simulink model "Due_Test"  (R2020a)
settings: Solver=FixedStepAuto  StartTime=0.0  StopTime=inf  FixedStep=T  RelTol=1e-3  EnableMultiTasking=on
undefined symbols (not defined in the file): Iumax, T, wmax
libraries: arduinolib x6, eeStairGenerator x1
settings Model: SILPILModeSetting=veronly  ExtModeTrigDuration=2  Creator=Nguyen Tung  LastModifiedBy=Nguyen Tung
settings OptimizationCC: StrengthReduction=on  PassReuseOutputArgsAs=Individual arguments  ZeroExternalMemoryAtStartup=off  ZeroInternalMemoryAtStartup=off  MaxStackSize=64  OptimizeBlockOrder=speed  OptimizationPriority=Speed  OptimizationCustomize=off  MultiThreadedLoops=on  EfficientTunableParamExpr=on
settings DebuggingCC: ParameterTunabilityLossMsg=error
settings HardwareCC: ProdBitPerPointer=32  ProdBitPerSizeT=32  ProdBitPerPtrDiffT=32  ProdLargestAtomicInteger=Long  ProdLargestAtomicFloat=Double  ProdWordSize=32  ProdHWDeviceType=ARM Compatible->ARM Cortex
settings SFSimCC: MATLABDynamicMemAlloc=off
settings RTWCC: SystemTargetFile=ert.tlc  HardwareBoard=Arduino Due  TLCOptions=-aInlineSetEventsForThisBaseRateFcn=TLC_FALSE -aSuppressMultiTaskScheduler=TLC_FALSE -aRateBasedStepFcn=1  TemplateMakefile=ert_default_tmf  GenerateReport=on  Toolchain=Arduino ARM  BuildConfiguration=Faster Runs
settings CodeAppCC: ForceParamTrailComments=on  IgnoreCustomStorageClasses=off  OperatorAnnotations=on  SimulinkDataObjDesc=on  SFDataObjDesc=on  InsertBlockDesc=on
settings ERTTargetCC: SupportContinuousTime=on  SupportVariableSizeSignals=on  ExtModeStaticAllocSize=20000

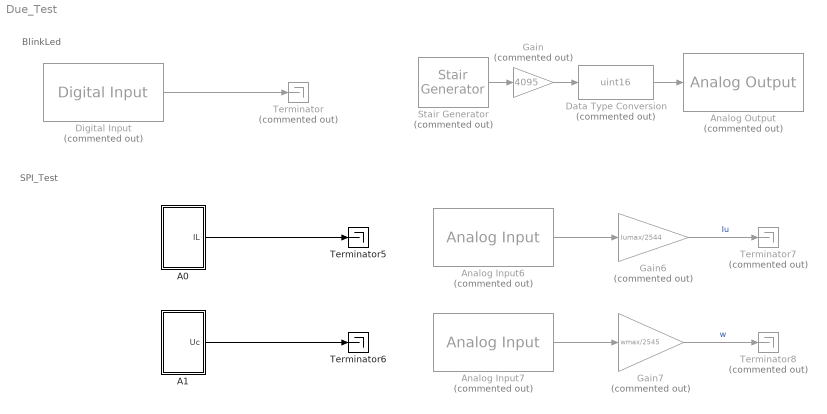
== system Due_Test ==
  note: SPI_Test
  note: BlinkLed
  A0 : Subsystem
  A1 : Subsystem
  Analog Input6 : arduinolib/Analog Input  Commented=on  pinNumber=2  ReadResultsOnly=off  ConversionTriggerSource=Software  ExternalTriggerType=uint32( 0 )  OutputDataType=uint16  EnableConversionCompleteNotify=off  EnableOuputStatus=off  SampleTime=T  blockPlatform=arduino
  Analog Input7 : arduinolib/Analog Input  Commented=on  pinNumber=3  ReadResultsOnly=off  ConversionTriggerSource=Software  ExternalTriggerType=uint32( 0 )  OutputDataType=uint16  EnableConversionCompleteNotify=off  EnableOuputStatus=off  SampleTime=T  blockPlatform=arduino
  Analog Output : arduinolib/Analog Output  Commented=on  DACpin=DAC1  blockPlatform=arduino
      settings: SourceProductBaseCode=ARDUINO
  Data Type Conversion : DataTypeConversion  Commented=on  OutDataTypeStr=uint16
  Digital Input : arduinolib/Digital Input  Commented=on  pinNumber=8  Direction=input  SampleTime=T  blockPlatform=arduino
  Gain : Gain  Commented=on  Gain=4095
  Gain6 : Gain  Commented=on  Gain=Iumax/2544
  Gain7 : Gain  Commented=on  Gain=wmax/2545
  Stair Generator : eeStairGenerator/Stair Generator  Commented=on  LabelModeActiveChoice=Discrete  TimeInput=[5 10 15 20 25 30 35]  AmplitudeInput=[0 0.2 0.4 0.6 0.8 1 0]  SampleTime=T  RepeatPattern=on  OutDataTypeStr=double
      settings: SourceProductBaseCode=PS
  Terminator : Terminator  Commented=on
  Terminator5 : Terminator
  Terminator6 : Terminator
  Terminator7 : Terminator  Commented=on
  Terminator8 : Terminator  Commented=on
  wires:
  Digital Input/1 -> Terminator/1
  Gain7/1 -> Terminator8/1  "w"
  Gain6/1 -> Terminator7/1  "Iu"
  Analog Input7/1 -> Gain7/1
  Analog Input6/1 -> Gain6/1
  Stair Generator/1 -> Gain/1
  Data Type Conversion/1 -> Analog Output/1
  Gain/1 -> Data Type Conversion/1
  A0/1(IL) -> Terminator5/1
  A1/1(Uc) -> Terminator6/1

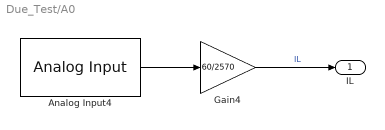
== system Due_Test/A0 ==
  Analog Input4 : arduinolib/Analog Input  pinNumber=0  ReadResultsOnly=off  ConversionTriggerSource=Software  ExternalTriggerType=uint32( 0 )  OutputDataType=uint16  EnableConversionCompleteNotify=off  EnableOuputStatus=off  SampleTime=T  blockPlatform=arduino
  Gain4 : Gain  Gain=60/2570
  IL : Outport
  wires:
  Analog Input4/1 -> Gain4/1
  Gain4/1 -> IL/1  "IL"

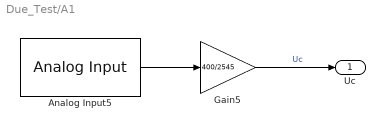
== system Due_Test/A1 ==
  Analog Input5 : arduinolib/Analog Input  pinNumber=1  ReadResultsOnly=off  ConversionTriggerSource=Software  ExternalTriggerType=uint32( 0 )  OutputDataType=uint16  EnableConversionCompleteNotify=off  EnableOuputStatus=off  SampleTime=T  blockPlatform=arduino
  Gain5 : Gain  Gain=400/2545
  Uc : Outport
  wires:
  Analog Input5/1 -> Gain5/1
  Gain5/1 -> Uc/1  "Uc"
